simulink model "PSO_controller2"  (R2020a)
settings: Solver=FixedStepAuto  StartTime=0.0  StopTime=Inf  RelTol=1e-3  EnableMultiTasking=on
libraries: c280xlib x11, c2837xDlib x4
settings Model: SimulationMode=external  ExtModeTrigDuration=8  Creator=Jason  LastModifiedBy=Jason
settings SolverCC: AutoInsertRateTranBlk=on
settings OptimizationCC: DefaultUnderspecifiedDataType=single  EnhancedBackFolding=on  PassReuseOutputArgsAs=Individual arguments  MaxStackSize=1024  OptimizeBlockOrder=speed  DifferentSizesBufferReuse=on  OptimizationCustomize=off  DenormalBehavior=FlushToZero  EfficientTunableParamExpr=on
settings DebuggingCC: ParameterTunabilityLossMsg=error
settings HardwareCC: ProdBitPerChar=16  ProdBitPerInt=16  ProdBitPerPointer=32  ProdBitPerSizeT=32  ProdBitPerPtrDiffT=32  ProdLargestAtomicInteger=Integer  ProdLargestAtomicFloat=None  ProdWordSize=16  ProdLongLongMode=on  ProdHWDeviceType=Texas Instruments->C2000
settings RTWCC: SystemTargetFile=ert.tlc  HardwareBoard=TI Delfino F28379D LaunchPad  TLCOptions=-aInlineSetEventsForThisBaseRateFcn=TLC_FALSE -aSuppressMultiTaskScheduler=TLC_FALSE -aRateBasedStepFcn=1  TemplateMakefile=ert_default_tmf  Toolchain=Texas Instruments Code Composer Studio (C2000)
settings CodeAppCC: ForceParamTrailComments=on  IgnoreCustomStorageClasses=off  OperatorAnnotations=on  SimulinkDataObjDesc=on  SFDataObjDesc=on  InsertBlockDesc=on
settings ERTTargetCC: TargetLangStandard=C99 (ISO)  CodeReplacementLibrary=TI C28x  DynamicStringBufferSize=401  SupportVariableSizeSignals=on  ExtModeStaticAllocSize=10000

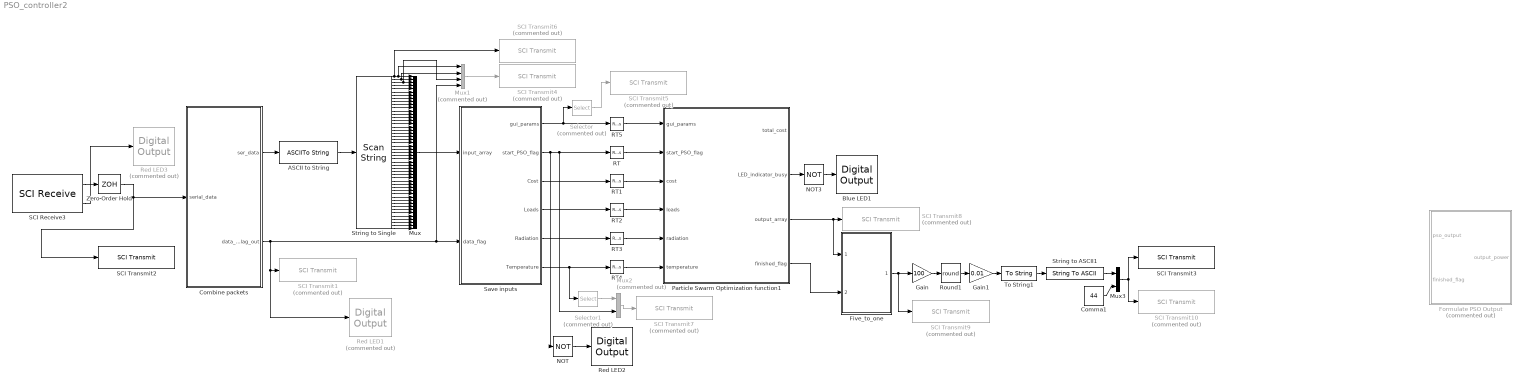
== system PSO_controller2 ==
  ASCII to String : ASCIIToString
  Blue LED1 : c2837xDlib/Digital Output  GPIO_Number=GPIO24~GPIO31  GPIO_Bit0=off  GPIO_BIT0_Toggle=off  GPIO_Bit1=off  GPIO_BIT1_Toggle=off  GPIO_Bit2=off  GPIO_BIT2_Toggle=off  GPIO_Bit3=off  GPIO_BIT3_Toggle=off  GPIO_Bit4=off  GPIO_BIT4_Toggle=off  GPIO_Bit5=off  GPIO_BIT5_Toggle=off  GPIO_Bit6=off  GPIO_BIT6_Toggle=off  GPIO_Bit7=on  GPIO_BIT7_Toggle=off
      settings: SourceProductBaseCode=TIC2000
  Combine packets : MATLAB Function  TreatAsAtomicUnit=on
  Comma1 : Constant  Value=44  OutDataTypeStr=uint8  SampleTime=-1
  Five_to_one : MATLAB Function  TreatAsAtomicUnit=on
  Formulate PSO Output : MATLAB Function  Commented=on  TreatAsAtomicUnit=on
  Gain : Gain  Gain=100
  Gain1 : Gain  Gain=0.01
  Mux : Mux  Inputs=49
  Mux1 : Mux  Commented=on
  Mux2 : Mux  Commented=on  Inputs=2
  Mux3 : Mux  Inputs=2
  NOT : Logic  Operator=NOT  IconShape=distinctive  AllPortsSameDT=off  OutDataTypeStr=boolean
  NOT3 : Logic  Operator=NOT  IconShape=distinctive  AllPortsSameDT=off  OutDataTypeStr=boolean
  Particle Swarm Optimization function1 : MATLAB Function  TreatAsAtomicUnit=on
  RT{,1..5} (6 alike) : RateTransition  OutPortSampleTime=0.1
  Red LED1 : c2837xDlib/Digital Output  Commented=on  GPIO_Number=GPIO32~GPIO39  GPIO_Bit0=off  GPIO_BIT0_Toggle=off  GPIO_Bit1=off  GPIO_BIT1_Toggle=off  GPIO_Bit2=on  GPIO_BIT2_Toggle=off  GPIO_Bit3=off  GPIO_BIT3_Toggle=off  GPIO_Bit4=off  GPIO_BIT4_Toggle=off  GPIO_Bit5=off  GPIO_BIT5_Toggle=off  GPIO_Bit6=off  GPIO_BIT6_Toggle=off  GPIO_Bit7=off  GPIO_BIT7_Toggle=off
      settings: SourceProductBaseCode=TIC2000
  Red LED2 : c2837xDlib/Digital Output  GPIO_Number=GPIO32~GPIO39  GPIO_Bit0=off  GPIO_BIT0_Toggle=off  GPIO_Bit1=off  GPIO_BIT1_Toggle=off  GPIO_Bit2=on  GPIO_BIT2_Toggle=off  GPIO_Bit3=off  GPIO_BIT3_Toggle=off  GPIO_Bit4=off  GPIO_BIT4_Toggle=off  GPIO_Bit5=off  GPIO_BIT5_Toggle=off  GPIO_Bit6=off  GPIO_BIT6_Toggle=off  GPIO_Bit7=off  GPIO_BIT7_Toggle=off
      settings: SourceProductBaseCode=TIC2000
  Red LED3 : c2837xDlib/Digital Output  Commented=on  GPIO_Number=GPIO32~GPIO39  GPIO_Bit0=off  GPIO_BIT0_Toggle=off  GPIO_Bit1=off  GPIO_BIT1_Toggle=off  GPIO_Bit2=on  GPIO_BIT2_Toggle=off  GPIO_Bit3=off  GPIO_BIT3_Toggle=off  GPIO_Bit4=off  GPIO_BIT4_Toggle=off  GPIO_Bit5=off  GPIO_BIT5_Toggle=off  GPIO_Bit6=off  GPIO_BIT6_Toggle=off  GPIO_Bit7=off  GPIO_BIT7_Toggle=off
      settings: SourceProductBaseCode=TIC2000
  Round1 : Rounding  Operator=round
  SCI Receive3 : c280xlib/SCI Receive  sciModule=B  dataHead=''  dataTail=''  dataType=uint8  dataDim=11  initValue=49  errOption=Output the last received value  errValue=0  sampleTime=0.005  outputStatus=on  postInterrupt=off  numFifo=1
      settings: SourceProductBaseCode=TIC2000
  SCI Transmit{1,4..10} (8 alike) : c280xlib/SCI Transmit  Commented=on  sciModule=A  dataHead=''  dataTail=''  postInterrupt=off  numFifo=1
  SCI Transmit2 : c280xlib/SCI Transmit  sciModule=A  dataHead=''  dataTail=''  postInterrupt=off  numFifo=1
  SCI Transmit3 : c280xlib/SCI Transmit  sciModule=B  dataHead=''  dataTail=''  postInterrupt=off  numFifo=1
  Save inputs : MATLAB Function  TreatAsAtomicUnit=on
  Selector : Selector  Commented=on  InputPortWidth=35  IndexOptions=Index vector (dialog)  Indices=[1:4]  OutputSizes=1
  Selector1 : Selector  Commented=on  InputPortWidth=49  IndexOptions=Index vector (dialog)  Indices=[1:3]  OutputSizes=1
  String to ASCII1 : StringToASCII  OutputVectorSize=9
  String to Single : ScanString  Format="\"ff%f,%f,%f,%f,%f,%f,%f,%f,%f,%f,%f,%f,%f,%f,%f,%f,%f,%f,%f,%f,%f,%f,%f,%f,%f,%f,%f,%f,%f,%f,%f,%f,%f,%f,%f,%f,%f,%f,%f,%f,%f,%f,%f,%f,%f,%f,%f,%f,%fE\""
  To String1 : ToString
  Zero-Order Hold : ZeroOrderHold  SampleTime=0.1
  wires:
  SCI Receive3/1 -> Zero-Order Hold/1
  Zero-Order Hold/1 -> Combine packets/1(serial_data), SCI Transmit2/1
  ASCII to String/1 -> String to Single/1
  String to Single/1 -> SCI Transmit6/1, Mux1/1, Mux/1
  String to Single/2 -> Mux1/2, Mux/2
  String to Single/3 -> Mux1/3, Mux/3
  String to Single/4 -> Mux/4
  String to Single/5 -> Mux/5
  String to Single/6 -> Mux/6
  String to Single/7 -> Mux/7
  String to Single/8 -> Mux/8
  String to Single/9 -> Mux/9
  String to Single/10 -> Mux/10
  String to Single/11 -> Mux/11
  String to Single/12 -> Mux/12
  String to Single/13 -> Mux/13
  String to Single/14 -> Mux/14
  String to Single/15 -> Mux/15
  String to Single/16 -> Mux/16
  String to Single/17 -> Mux/17
  String to Single/18 -> Mux/18
  String to Single/19 -> Mux/19
  String to Single/20 -> Mux/20
  String to Single/21 -> Mux/21
  String to Single/22 -> Mux/22
  String to Single/23 -> Mux/23
  String to Single/24 -> Mux/24
  String to Single/25 -> Mux/25
  String to Single/26 -> Mux/26
  String to Single/27 -> Mux/27
  String to Single/28 -> Mux/28
  String to Single/29 -> Mux/29
  String to Single/30 -> Mux/30
  String to Single/31 -> Mux/31
  String to Single/32 -> Mux/32
  String to Single/33 -> Mux/33
  String to Single/34 -> Mux/34
  String to Single/35 -> Mux/35
  String to Single/36 -> Mux/36
  String to Single/37 -> Mux/37
  String to Single/38 -> Mux/38
  String to Single/39 -> Mux/39
  String to Single/40 -> Mux/40
  String to Single/41 -> Mux/41
  String to Single/42 -> Mux/42
  String to Single/43 -> Mux/43
  String to Single/44 -> Mux/44
  String to Single/45 -> Mux/45
  String to Single/46 -> Mux/46
  String to Single/47 -> Mux/47
  String to Single/48 -> Mux/48
  String to Single/49 -> Mux/49
  Mux/1 -> Save inputs/1(input_array)
  Particle Swarm Optimization function1/2(LED_indicator_busy) -> NOT3/1
  NOT3/1 -> Blue LED1/1
  Save inputs/2(start_PSO_flag) -> NOT/1, Mux2/2, RT/1
  Save inputs/3(Cost) -> RT1/1
  Save inputs/4(Loads) -> RT2/1
  Save inputs/5(Radiation) -> RT3/1
  Save inputs/6(Temperature) -> RT4/1, Selector1/1
  SCI Receive3/2 -> Red LED3/1
  Save inputs/1(gui_params) -> Selector/1, RT5/1
  RT5/1 -> Particle Swarm Optimization function1/1(gui_params)
  RT/1 -> Particle Swarm Optimization function1/2(start_PSO_flag)
  RT1/1 -> Particle Swarm Optimization function1/3(cost)
  RT2/1 -> Particle Swarm Optimization function1/4(loads)
  RT3/1 -> Particle Swarm Optimization function1/5(radiation)
  RT4/1 -> Particle Swarm Optimization function1/6(temperature)
  Mux3/1 -> SCI Transmit3/1, SCI Transmit10/1
  Particle Swarm Optimization function1/3(output_array) -> SCI Transmit8/1, Five_to_one/1(input_array_five)
  Combine packets/2(data_status_flag_out) -> Mux1/4, Save inputs/2(data_flag), Red LED1/1, SCI Transmit1/1
  Combine packets/1(ser_data) -> ASCII to String/1
  Mux1/1 -> SCI Transmit4/1
  Selector/1 -> SCI Transmit5/1
  Selector1/1 -> Mux2/1
  Mux2/1 -> SCI Transmit7/1
  Particle Swarm Optimization function1/4(finished_flag) -> Five_to_one/2(finished_flag)
  Gain/1 -> Round1/1
  Five_to_one/1(out_array_one) -> Gain/1, SCI Transmit9/1
  Round1/1 -> Gain1/1
  Gain1/1 -> To String1/1
  To String1/1 -> String to ASCII1/1
  Comma1/1 -> Mux3/2
  String to ASCII1/1 -> Mux3/1
  NOT/1 -> Red LED2/1

== matlab function PSO_controller2/Particle Swarm Optimization function1 ==
  data: total_cost output; gui_params input; start_PSO_flag input; cost input; LED_indicator_busy output; output_array output; loads input; finished_flag output; radiation input; temperature input
% function [total_cost,LED_indicator_busy,output_array,output_array_full,finished_flag,part_table]  = ParticleSwarm_algorithm(gui_params,start_PSO_flag,cost,loads,radiation,temperature)
function [total_cost,LED_indicator_busy,output_array,finished_flag]  = ParticleSwarm_algorithm(gui_params,start_PSO_flag,cost,loads,radiation,temperature)

persistent numParticles maxEpochs currentEpoch currentPar particlesTable neighborIndex EV_bat_n SoC_initial_ev dt Ev_bat_capacity SoC_target_ev Tmax ...
    Tmin T_in_initial V C rho Uwall Uwindow Fwall Fwindow aw Rsej taf_window SC QEC_max QEC_min COP SOC_EV_penalty_multiplier SOC_EV_target_penalty_multiplier ...
    PPEV_diff_penalty_multiplier offset_variable partial_cost_multiplier SoCmax_ev SoCmin_ev lb ub Pmin_ev Pmax_ev Pmax_bat Pmin_bat SoC_initial_bat ...
    SoC_target_bat SoCmax_bat SoCmin_bat bat_capacity bat_n span CostOfPower cSelf cSocial inertia outdoor_temperature solar_radiation heatcool_sign Zeta Qin Qsw Qsg ...
    QEC_diff_penalty_multiplier Tin_penalty_multiplier T t LED_indicator_flag dim1 dim2 dim3 dim4 numVariables tfInvalidMask SOC_bat_penalty_multiplier PBAT_diff_penalty_multiplier home_load ...
    LOAD_equals_penalty_multiplier penaltiesTable minNeighborhoodSize maxParticles maxDimensions output_counter output_delay;



maxParticles = 10;
% maxParticles = 3;
maxDimensions = 13+13+13+13;

% assert(maxEpochs<=1000)

if isempty(LED_indicator_flag)
    LED_indicator_flag = 0;
end


%% Case 1: First run of function, initialize variables
if isempty(currentEpoch)
    
    %     rng shuffle       %MAY NEED TO BE REMOVED
    
    T = 24;
    heatcool_sign = -1;
    output_delay = 1;
    
    % minNeighborhoodSize = max(2,floor(numParticles*0.25)); %0.25 =Minimum adaptive neighborhood size, a scalar from 0 to 1. Default is 0.25.
    minNeighborhoodSize = 2;
    
    
    CostOfPower = single(zeros(1,49));
    home_load = single(zeros(1,49));
    solar_radiation = single(zeros(1,49));
    outdoor_temperature = single(zeros(1,49));

    SOC_EV_penalty_multiplier = 0.5;
    SOC_EV_target_penalty_multiplier = 1.5;
%     PPEV_diff_penalty_multiplier = 0.001;
    PPEV_diff_penalty_multiplier = 0.005;
    
    SOC_bat_penalty_multiplier = 1;
    PBAT_diff_penalty_multiplier = 0.005;
    
    QEC_diff_penalty_multiplier = 0;  % Penalty for large deviations of the QEC
    Tin_penalty_multiplier = 0.6; % Penalty for not maintaining the internal temperature between the desired limits
    
    LOAD_equals_penalty_multiplier = 1; % Penalty for the initial and load shifted loads not having equal sums
    
    offset_variable = 0; %Offset the sum of power rates to avoid reaching negative values
    partial_cost_multiplier = 4;
    cSelf = single(1.496);
    cSocial = single(1.496);
    inertia = single(0.4);%TODO: make inertia vector for each variable
    
    currentEpoch = single(0);
    currentPar = single(0);
    
    
    
    %% Initializations
    numParticles = single(1);
    maxEpochs = single(1);
    
    dt = single(0.5);
    dim1 = single(0);  %EV PSO dimensions
    dim2 = single(0);  %Thermal PSO dimensions
    dim3 = single(0);  %BAT PSO dimensions
    dim4 = single(0);   %Load shifting dimensions
    Pmax_ev = single(0);
    Pmin_ev = single(0);
    EV_bat_n = single(0);
    SoC_initial_ev = single(0);
    SoC_target_ev = single(0);
    Pmax_bat = single(0);
    Pmin_bat = single(0);
    SoC_initial_bat = single(0);
    SoC_target_bat = single(0);
    bat_capacity = single(0);
    bat_n = single(0);
    Tmax = single(0);
    Tmin = single(0);
    T_in_initial = single(0);
    V = single(0);
    C = single(0);
    rho = single(0);
    Uwall = single(0);
    Uwindow = single(0);
    Fwall = single(0);
    Fwindow = single(0);
    aw = single(0);
    Rsej = single(0);
    taf_window = single(0);
    SC = single(0);
    QEC_max = single(0);
    QEC_min = single(0);
    COP = single(0);
    Ev_bat_capacity = single(0);
    t = single(linspace(0,24,(24/0.5)+1));
    
    numVariables = single(maxDimensions);
    tfInvalidMask = single(zeros(10,3*52+1));
    
    Zeta = single((rho*C*V)/(0.5*3600));     %dt is converted to seconds in order to match the rest of the units
    Qin = single(0.2*ones(1,49));
    Qsw = single(aw * Rsej * Uwall * Fwall * solar_radiation);
    Qsg = single(0.001*taf_window * SC * Fwindow * solar_radiation);
    
    SoCmax_ev = single(Ev_bat_capacity*0.9);
    SoCmin_ev = single(Ev_bat_capacity*0.1);
    SoCmax_bat = single(bat_capacity*0.9);
    SoCmin_bat = single(bat_capacity*0.1);
    
    lb = single(zeros(1,maxDimensions));
    ub = single(zeros(1,maxDimensions));
    %     span = single(ub - lb);
    particlesTable = single(zeros(uint8(maxParticles),3*uint8(maxDimensions+1))); %set particlesTable to the largest array size
    output_counter = single(1);
    
    
end

%     %debug
%
%
%     total_cost = 0;
%     LED_indicator_busy = 0;
%     finished_flag = 0;
%     output_array = single(-1*ones(1,4));
%
%
%     %debug

%% Case 2.1: Start optimization (once data has been received), read data and set initial values
if currentEpoch == 0 && start_PSO_flag == 1
    
    
    
    numParticles = gui_params(1);
    maxEpochs = gui_params(2);
    assert(numParticles<=maxParticles)        %Particle matrix will be too big if its more than 11
    
    dim1 = gui_params(3);  %EV PSO dimensions
    dim2 = gui_params(4);  %Thermal PSO dimensions
    dim3 = gui_params(5);  %BAT PSO dimensions
    dim4 = gui_params(6);   %Load shifting dimensions
    assert(dim1<14)
    assert(dim2<14)
    assert(dim3<14)
    assert(dim4<14)
    
    Pmax_ev = gui_params(7);
    Pmin_ev = gui_params(8);
    EV_bat_n = gui_params(9);
    SoC_initial_ev = gui_params(10);
    SoC_target_ev = gui_params(11);
    Pmax_bat = gui_params(12);
    Pmin_bat = gui_params(13);
    SoC_initial_bat = gui_params(14);
    SoC_target_bat = gui_params(15);
    bat_capacity = gui_params(16);
    bat_n = gui_params(17);
    Tmax = gui_params(18);
    Tmin = gui_params(19);
    T_in_initial = gui_params(20);
    V = gui_params(21);
    C = gui_params(22);
    rho = gui_params(23);
    Uwall = gui_params(24);
    Uwindow = gui_params(25);
    Fwall = gui_params(26);
    Fwindow = gui_params(27);
    aw = gui_params(28);
    Rsej = gui_params(29);
    taf_window = gui_params(30);
    SC = gui_params(31);
    QEC_max = gui_params(32);
    QEC_min = gui_params(33);
    COP = gui_params(34);
    Ev_bat_capacity = gui_params(35);
    
    CostOfPower(1:49) = cost(1:49);
    home_load(1:49) = loads(1:49);
    solar_radiation(1:49) = radiation(1:49);
    outdoor_temperature(1:49) = temperature(1:49);
    
    t = single(0:dt:T);
    numVariables = single(dim1+dim2+dim3+dim4);
    assert(numVariables <53)
    tfInvalidMask = single(zeros(numParticles,3*numVariables+1));
    
    Zeta = single((rho*C*V)/(dt*3600));     %dt is converted to seconds in order to match the rest of the units
    Qin = single(0.2*ones(1,length(t)));
    Qsw = single(aw * Rsej * Uwall * Fwall * solar_radiation);
    Qsg = single(0.001*taf_window * SC * Fwindow * solar_radiation);
    
    SoCmax_ev = single(Ev_bat_capacity*0.9);
    SoCmin_ev = single(Ev_bat_capacity*0.1);
    SoCmax_bat = single(bat_capacity*0.9);
    SoCmin_bat = single(bat_capacity*0.1);
    
    Load_shifting_min = 0.7;
    Load_shifting_max = 1.3;
    
    
    
    if QEC_min == 0 && QEC_max == 0     %No heat system or load system
        QEC_diff_penalty_multiplier = 0;
        Tin_penalty_multiplier = 0;
        LOAD_equals_penalty_multiplier = 0;
        Load_shifting_min = 0;
        Load_shifting_max = 0;
    end
    
    
    lb = single([Pmin_ev*ones(1,dim1) QEC_min*ones(1,dim2) Pmin_bat*ones(1,dim3) Load_shifting_min*ones(1,dim4)]);
    ub = single([Pmax_ev*ones(1,dim1) QEC_max*ones(1,dim2) Pmax_bat*ones(1,dim3) Load_shifting_max*ones(1,dim4)]);
    span = single(ub - lb);
    
    %     particlesTable = single(zeros(uint8(numParticles),3*uint8(numVariables+1))); %kathe numVariables plithos timon, gia kathe dianusma (current pos, best pos, velocity)
    particlesTable(:,1:numVariables) = repmat(lb,numParticles,1) + repmat(span,numParticles,1) .* rand(numParticles,numVariables);
    particlesTable(:,numVariables+2:numVariables+2+numVariables-1) = particlesTable(:,1:numVariables);
    % Initialize velocities by randomly sampling over the smaller of options.InitialSwarmSpan or ub-lb. Note that min will be InitialSwarmSpan if either lb or ub is not finite.
    vmax = single(span);
    particlesTable(:,2*numVariables+2:2*numVariables+2+numVariables-1) = repmat(-vmax,numParticles,1) + ...
        repmat(2*vmax,numParticles,1) .* rand(numParticles,numVariables);
    
    currentPar = currentPar + 1;
    
    % EV Calculations
    [PPEV,state_of_charge_ev] = EV_Calculations(dt,T,dim1,currentPar,particlesTable,EV_bat_n,SoC_initial_ev);
    
    % Heat System Calculations
    [QEC,indoor_temperature] = Thermal_Calculations(dt,T,dim1,dim2,currentPar,particlesTable,COP,T_in_initial,heatcool_sign,Zeta,Uwall,Uwindow,Fwall,Fwindow,outdoor_temperature,Qin,Qsw,Qsg);
    
    % BAT Calculations
    [PBAT,state_of_charge_bat] = Bat_Calculations(dt,T,dim1,dim2,dim3,currentPar,particlesTable,bat_n,SoC_initial_bat);
    
    % LOAD Calculations
    [PLOAD] = Load_Calculations(dt,T,dim1,dim2,dim3,dim4,currentPar,particlesTable,home_load);
    
    % EV Penalty
    [SOC_ev_penalty,SOC_ev_target_penalty,PPEV_diff_penalty] = EV_Penalties(state_of_charge_ev,SoCmax_ev,SoCmin_ev,PPEV,SoC_target_ev) ;
    
    % Heat System Penalty
    [Tin_penalty,QEC_diff_penalty] = Thermal_Penalties(QEC,indoor_temperature,Tmax,Tmin);
    
    % BAT Penalty
    [SOC_bat_penalty,PBAT_diff_penalty] = Bat_Penalties(state_of_charge_bat,SoCmax_bat,SoCmin_bat,PBAT,SoC_target_bat) ;
    
    % LOAD penalty
    [Load_equals_penalty] = Load_Penalties(PLOAD,home_load);
    
    % Cost Calculations
    cost_partial = single(sum((PPEV+abs(QEC)+PBAT+PLOAD').*CostOfPower)*dt);
    total_cost =single((SOC_EV_target_penalty_multiplier * SOC_ev_target_penalty + SOC_EV_penalty_multiplier * SOC_ev_penalty + ...
        PPEV_diff_penalty_multiplier * PPEV_diff_penalty + QEC_diff_penalty_multiplier*QEC_diff_penalty + Tin_penalty_multiplier*Tin_penalty + ...
        SOC_bat_penalty * SOC_bat_penalty_multiplier + PBAT_diff_penalty * PBAT_diff_penalty_multiplier + Load_equals_penalty * LOAD_equals_penalty_multiplier)+ ...
        (partial_cost_multiplier*(offset_variable+cost_partial)));
    
    particlesTable(currentPar,numVariables+1) = total_cost; %fval of previous particle stored as the best value of this particle (since it is the first time that it gets a value)
    

    
    %Finalize initialization, start main loop
    if currentPar == numParticles
        currentEpoch =single(1);
        currentPar = single(0);
        
    end
    
    LED_indicator_busy = 0;
    finished_flag = single(0);

    output_array = single(-1*ones(1,5));
    output_array(1) = currentPar;
    output_array(2) = numParticles;
    output_array(3) = maxEpochs;
    output_array(4) = dim1;
    output_array(5) = dim2;
    
    %% Case 2.2: Main loop of optimization
elseif currentEpoch <= maxEpochs && start_PSO_flag == 1
    
    
    
    if LED_indicator_flag == 0
        LED_indicator_flag = 1;
        LED_indicator_busy = 1;
    else
        LED_indicator_flag = 0;
        LED_indicator_busy = 0;
    end
    
    currentPar = currentPar + 1;
    
    %     part_table = particlesTable(currentPar,1:157)';
    %     part_table(1)=single(222222);
    %     part_table(2)=particlesTable(currentPar,53);
    
    if currentPar == 1
        
        % Generate a random neighborhood for each particle that includes the particle itself
        neighborIndex = zeros(numParticles, minNeighborhoodSize);
        neighborIndex(:, 1) = 1:numParticles; % First neighbor is self
        for i = 1:numParticles
            % Determine random neighbors that exclude the particle itself, which is (numParticles-1) particles
            neighbors = randperm(numParticles-1, minNeighborhoodSize-1);
            % Add 1 to indices that are >= current particle index
            iShift = neighbors >= i;
            neighbors(iShift) = neighbors(iShift) + 1;
            neighborIndex(i,2:end) = neighbors;
        end
        
        randSelf = rand(numParticles, numVariables);
        randSocial = rand(numParticles, numVariables);
        
        % Update the velocities
        
        temp1 = inertia*particlesTable(:,2*numVariables+2:2*numVariables+2+numVariables-1);
        temp2 = cSelf*randSelf.*(particlesTable(:,numVariables+2:numVariables+2+numVariables-1)-particlesTable(:,1:numVariables));
        %  temp3 =  cSocial*randSocial.*(particlesTable(bestNeighborIndex,numVariables+2:numVariables+2+numVariables-1)-particlesTable(:,1:numVariables))
        
        temp3 =  cSocial*randSocial.*(particlesTable(neighborIndex(:,2:end),numVariables+2:numVariables+2+numVariables-1)-particlesTable(:,1:numVariables));
        newVelocities =  temp1 + ...
            temp2 + ... %%thesi poy eixe kaluteri timi - current thesi
            temp3;
        
        particlesTable(:,2*numVariables+2:2*numVariables+2+numVariables-1) = newVelocities;
        
        % Update the positions
        newPopulation = particlesTable(:,1:numVariables) + particlesTable(:,2*numVariables+2:2*numVariables+2+numVariables-1);
        
        tfInvalid=zeros(numParticles,numVariables);
        for i=1:numParticles
            tfInvalid(i,:) = newPopulation(i,:) < lb;
        end
        tfInvalidMask(:,2*numVariables+2:end) = tfInvalid;
        mask = (tfInvalidMask==1);
        
        
        if any(any(tfInvalid))
            for y=1:numVariables
                for i=1:numParticles
                    if tfInvalid(i,y)==1
                        newPopulation(i,y)= lb(y);
                    end
                end
            end
            particlesTable(mask) = 0;
        end
        
        
        tfInvalid=zeros(numParticles,numVariables);
        for i=1:numParticles
            tfInvalid(i,:) = newPopulation(i,:) > ub;
        end
        tfInvalidMask(:,2*numVariables+2:end) = tfInvalid;
        mask = (tfInvalidMask==1);
        if any(any(tfInvalid))
            for y=1:numVariables
                for i=1:numParticles
                    if tfInvalid(i,y)==1
                        newPopulation(i,y)= ub(y);
                    end
                end
            end
            particlesTable(mask) = 0;
        end
        particlesTable(:,1:numVariables) = newPopulation;
    end
    
    %     part_table(3)=particlesTable(currentPar,53);
    
    
    % EV Calculations
    [PPEV,state_of_charge_ev] = EV_Calculations(dt,T,dim1,currentPar,particlesTable,EV_bat_n,SoC_initial_ev);
    
    % Thermal Calculations
    [QEC,indoor_temperature] = Thermal_Calculations(dt,T,dim1,dim2,currentPar,particlesTable,COP,T_in_initial,heatcool_sign,Zeta,Uwall,Uwindow,Fwall,Fwindow,outdoor_temperature,Qin,Qsw,Qsg);
    
    % BAT Calculations
    [PBAT,state_of_charge_bat] = Bat_Calculations(dt,T,dim1,dim2,dim3,currentPar,particlesTable,bat_n,SoC_initial_bat);
    
    % LOAD Calculations
    [PLOAD] = Load_Calculations(dt,T,dim1,dim2,dim3,dim4,currentPar,particlesTable,home_load);
    
    % EV Penalty
    [SOC_ev_penalty,SOC_ev_target_penalty,PPEV_diff_penalty] = EV_Penalties(state_of_charge_ev,SoCmax_ev,SoCmin_ev,PPEV,SoC_target_ev) ;
    
    % Heat System Penalty
    [Tin_penalty,QEC_diff_penalty] = Thermal_Penalties(QEC,indoor_temperature,Tmax,Tmin);
    
    % BAT Penalty
    [SOC_bat_penalty,PBAT_diff_penalty] = Bat_Penalties(state_of_charge_bat,SoCmax_bat,SoCmin_bat,PBAT,SoC_target_bat) ;
    
    % LOAD penalty
    [Load_equals_penalty] = Load_Penalties(PLOAD,home_load);
    
    %% ------------- Cost Calculations -------------
    
    if QEC_min == 0 && QEC_max == 0     %No heat system or load system
        cost_partial = single(sum((PPEV+PBAT).*CostOfPower)*dt);
    else
        cost_partial = single(sum((PPEV+abs(QEC)+PBAT+PLOAD').*CostOfPower)*dt);
    end
    total_cost =single((SOC_EV_target_penalty_multiplier * SOC_ev_target_penalty + SOC_EV_penalty_multiplier * SOC_ev_penalty + ...
        PPEV_diff_penalty_multiplier * PPEV_diff_penalty + QEC_diff_penalty_multiplier*QEC_diff_penalty + Tin_penalty_multiplier*Tin_penalty + ...
        SOC_bat_penalty * SOC_bat_penalty_multiplier + PBAT_diff_penalty * PBAT_diff_penalty_multiplier + Load_equals_penalty * LOAD_equals_penalty_multiplier)+ ...
        (partial_cost_multiplier*(offset_variable+cost_partial)));
    
    %     part_table(4)=particlesTable(currentPar,53);
    %     part_table(5)=total_cost;
    
    
    if total_cost < particlesTable(currentPar,numVariables+1)
        
        particlesTable(currentPar,numVariables+1) = total_cost;
        particlesTable(currentPar,numVariables+2:numVariables+2+numVariables-1) = particlesTable(currentPar,1:numVariables);
        
        
        %         %DEBUGGING, REMOVE LATER
        %         penaltiesTable(currentPar,1) = SOC_EV_target_penalty_multiplier * SOC_ev_target_penalty;
        %         penaltiesTable(currentPar,2) = SOC_EV_penalty_multiplier * SOC_ev_penalty;
        %         penaltiesTable(currentPar,3) = PPEV_diff_penalty_multiplier * PPEV_diff_penalty;
        %         penaltiesTable(currentPar,4) = QEC_diff_penalty_multiplier*QEC_diff_penalty;
        %         penaltiesTable(currentPar,5) = Tin_penalty_multiplier*Tin_penalty;
        %         penaltiesTable(currentPar,6) = SOC_bat_penalty * SOC_bat_penalty_multiplier;
        %         penaltiesTable(currentPar,7) = PBAT_diff_penalty * PBAT_diff_penalty_multiplier;
        %         penaltiesTable(currentPar,8) = Load_equals_penalty * LOAD_equals_penalty_multiplier;
        %         penaltiesTable(currentPar,10) = cost_partial;
        %         penaltiesTable(currentPar,9)= (SOC_EV_target_penalty_multiplier * SOC_ev_target_penalty + SOC_EV_penalty_multiplier * SOC_ev_penalty + ...
        %         PPEV_diff_penalty_multiplier * PPEV_diff_penalty + QEC_diff_penalty_multiplier*QEC_diff_penalty + Tin_penalty_multiplier*Tin_penalty + ...
        %         SOC_bat_penalty * SOC_bat_penalty_multiplier + PBAT_diff_penalty * PBAT_diff_penalty_multiplier + Load_equals_penalty * LOAD_equals_penalty_multiplier);
        % %         penaltiesTable(10)= partial_cost_multiplier*(offset_variable+cost_partial);
        %
        %
    end
    
    %     part_table(6)=particlesTable(currentPar,53);
    %     part_table(7)=total_cost;
    
    output_array = single(-2*ones(1,5));
    
    finished_flag = single(0);
    %     part_table = particlesTable(currentPar,1:157)';
    
    %End of current epoch
    if currentPar == numParticles
        currentEpoch = currentEpoch + 1;
        
%         if currentEpoch > maxEpochs 
%             particlesTable(:,numVariables+2:numVariables+numVariables+1) = 100.*(particlesTable(:,numVariables+2:numVariables+numVariables+1));
%             particlesTable(:,numVariables+2:numVariables+numVariables+1) = round(particlesTable(:,numVariables+2:numVariables+numVariables+1));
%             particlesTable(:,numVariables+2:numVariables+numVariables+1) = (particlesTable(:,numVariables+2:numVariables+numVariables+1)/100);
%         end
        
        currentPar = single(0);
        return;
        %End of current particle
    elseif currentPar>=1 && currentPar<numParticles
        return;
    else %Should never reach here
        error('Particle Loop Error')
    end
    
    
    %% Case 2.3: Optimization ended, and no new data has been sent - Output power arrays
elseif start_PSO_flag == 1  %end of PSO calculations
    
    [total_cost,i_min_cost] = min(particlesTable(1:numParticles,numVariables+1));
    LED_indicator_busy = 1;
    
    finished_flag = single(1);
    
    %% ------------- Debug Calculations and plots -------------
    
    particlesTable(:,1:numVariables) = particlesTable(:,numVariables+2:numVariables+numVariables+1);
    
    
    [PPEV,state_of_charge_ev] = EV_Calculations(dt,T,dim1,i_min_cost,particlesTable,EV_bat_n,SoC_initial_ev);
    [QEC,indoor_temperature] = Thermal_Calculations(dt,T,dim1,dim2,i_min_cost,particlesTable,COP,T_in_initial,heatcool_sign,Zeta,Uwall,Uwindow,Fwall,Fwindow,outdoor_temperature,Qin,Qsw,Qsg);
    [PBAT,state_of_charge_bat] = Bat_Calculations(dt,T,dim1,dim2,dim3,i_min_cost,particlesTable,bat_n,SoC_initial_bat);
    [PLOAD] = Load_Calculations(dt,T,dim1,dim2,dim3,dim4,i_min_cost,particlesTable,home_load);
    
    PPEV(end)=0;
    PBAT(end)=0;
    
%     
    output_array_temp = single([1111111 PPEV(1:49) 2222222 PBAT(1:49) 3333333 QEC(1:49) 4444444 indoor_temperature(1:49) ...
        5555555 state_of_charge_ev(1:49) 6666666 state_of_charge_bat(1:49) 7777777 PLOAD(1:49)']);
%     debug_array = [1 2 3 4 5 6 7 8 9 10 11 12 13 14 15 16 17 18 19 20 21 22 23 24 25 26 27 28 29 30 31 32 33 34 35 36 37 38 39 40 41 42 43 44 45 46 47 48 49];
%     output_array_temp = single([1111111 debug_array 2222222 debug_array 3333333 debug_array 4444444 debug_array ...
%         5555555 debug_array 6666666 debug_array 7777777 debug_array]);
%     
    output_array = single(-4*ones(1,5));
    output_array(1) = output_array_temp(output_counter);
    output_array(2) = output_array_temp(output_counter+1);
    output_array(3) = output_array_temp(output_counter+2);
    output_array(4) = output_array_temp(output_counter+3);
    output_array(5) = output_array_temp(output_counter+4);
    
        output_delay = output_delay + 1;
        if output_delay > 5
            output_counter = output_counter + 5;
            output_delay = 1;
        end
    
%     output_counter = output_counter + 5;
    
    
    if output_counter > size(output_array_temp)
        output_counter = single(1);
    end
    
    
    %% Case 2.4: Optimization ended, new data is being sent
else
    total_cost = single(100000);
    LED_indicator_busy = 0;
    finished_flag = single(0);
    %     part_table = single(38*ones(1,157)');
    output_array = single(-3*ones(1,5));
    
    currentEpoch = single(0);
    
end

end



function [PPEV,state_of_charge_ev] = EV_Calculations(dt,T,dim1,currentPar,particlesTable,EV_bat_n,SoC_initial_ev)

PPEV_not_interp = single(particlesTable(currentPar,1:dim1));
% PPEV = single(interp1(linspace(0,T,dim1),PPEV_not_interp,linspace(0,T,(T/dt)+1),'spline'));
PPEV = single(interp1(0:2:T,PPEV_not_interp,0:0.5:T,'spline'));

PPEV_actual = single(zeros(1,length(PPEV))');
for z=1:length(PPEV_actual)
    if PPEV(z)>=0
        PPEV_actual(z)=PPEV(z)*EV_bat_n;
    else
        PPEV_actual(z)=PPEV(z)/EV_bat_n;
    end
end

state_of_charge_ev = single(zeros(1,length(PPEV)));
state_of_charge_ev(1)=SoC_initial_ev;
state_of_charge_ev(2:end)=SoC_initial_ev+cumsum(PPEV_actual(1:end-1))*dt;

end
function [QEC,indoor_temperature] = Thermal_Calculations(dt,T,dim1,dim2,currentPar,particlesTable,COP,T_in_initial,heatcool_sign,Zeta,Uwall,Uwindow,Fwall,Fwindow,outdoor_temperature,Qin,Qsw,Qsg)

QEC_not_interp = single(particlesTable(currentPar,dim1+1:dim1+dim2));  % TODO Fix number of variables once you add more power arrays to calculate
QEC = single(interp1(linspace(0,T,dim2),QEC_not_interp,linspace(0,T,(T/dt)+1),'spline'));
QEC_thermal = single(QEC*COP);

indoor_temperature=single(zeros(1,length(QEC_thermal)));
indoor_temperature(1) =T_in_initial;

for i=2:length(QEC)
    indoor_temperature(i) = indoor_temperature(i-1) + heatcool_sign*QEC_thermal(i-1)/Zeta + ...
        (Uwall*Fwall*(outdoor_temperature(i-1)-indoor_temperature(i-1))+ ...
        Uwindow*Fwindow*(outdoor_temperature(i-1)-indoor_temperature(i-1))+ ...
        Qin(i-1)+Qsw(i-1)+Qsg(i-1))/Zeta;
end

end
function [PBAT,state_of_charge_bat] = Bat_Calculations(dt,T,dim1,dim2,dim3,currentPar,particlesTable,bat_n,SoC_initial_bat)

PBAT_not_interp = single(particlesTable(currentPar,dim1+dim2+1:dim1+dim2+dim3));
PBAT = single(interp1(linspace(0,T,dim3),PBAT_not_interp,linspace(0,T,(T/dt)+1),'spline'));

PBAT_actual = zeros(1,length(PBAT))';
for z=1:length(PBAT_actual)
    if PBAT(z)>=0
        PBAT_actual(z)=PBAT(z)*bat_n;
    else
        PBAT_actual(z)=PBAT(z)/bat_n;
    end
end

state_of_charge_bat = single(zeros(1,length(PBAT)));
state_of_charge_bat(1)=SoC_initial_bat;
state_of_charge_bat(2:end) = SoC_initial_bat + cumsum(PBAT_actual(1:end-1))*dt;

end
function [PLOAD] = Load_Calculations(dt,T,dim1,dim2,dim3,dim4,currentPar,particlesTable,home_load)

PLOAD_shifting_not_interp = single(particlesTable(currentPar,dim1+dim2+dim3+1:dim1+dim2+dim3+dim4));
PLOAD_shifting = single(interp1(linspace(0,T,dim4),PLOAD_shifting_not_interp,linspace(0,T,(T/dt)+1),'spline'));
PLOAD = (PLOAD_shifting.*home_load)';

end
function [SOC_ev_penalty,SOC_ev_target_penalty,PPEV_diff_penalty] = EV_Penalties(state_of_charge_ev,SoCmax_ev,SoCmin_ev,PPEV,SoC_target_ev)
SOC_ev_penalty = single(0);
for i=1:length(state_of_charge_ev)
    if state_of_charge_ev(i)>SoCmax_ev
        SOC_ev_penalty = SOC_ev_penalty + (state_of_charge_ev(i) - SoCmax_ev);
    elseif  state_of_charge_ev(i)<SoCmin_ev
        SOC_ev_penalty = SOC_ev_penalty + (SoCmin_ev - state_of_charge_ev(i));
    end
end
SOC_ev_target_penalty= single(abs(state_of_charge_ev(end)-SoC_target_ev));

PPEV_diff_penalty = single(sum(abs(diff(PPEV))));
end
function [Tin_penalty,QEC_diff_penalty] = Thermal_Penalties(QEC,indoor_temperature,Tmax,Tmin)

Tin_penalty = single(0);
for i=1:length(QEC)
    if indoor_temperature(i)>Tmax(1)
        Tin_penalty = Tin_penalty + (indoor_temperature(i) - Tmax(1));
    elseif  indoor_temperature(i)<Tmin(1)
        Tin_penalty = Tin_penalty + (Tmin(1) - indoor_temperature(i));
    end
end
QEC_diff_penalty=single(sum(abs(diff(QEC))));
end
function [SOC_bat_penalty,PBAT_diff_penalty] = Bat_Penalties(state_of_charge_bat,SoCmax_bat,SoCmin_bat,PBAT,SoC_target_bat)
SOC_bat_penalty = single(0);
for i=1:length(PBAT)
    if state_of_charge_bat(i)>SoCmax_bat
        SOC_bat_penalty = SOC_bat_penalty + (state_of_charge_bat(i) - SoCmax_bat);
    elseif  state_of_charge_bat(i)<SoCmin_bat
        SOC_bat_penalty = SOC_bat_penalty + (SoCmin_bat - state_of_charge_bat(i));
    end
end
SOC_bat_penalty = SOC_bat_penalty + abs(state_of_charge_bat(end)-SoC_target_bat);
PBAT_diff_penalty=sum(abs(diff(PBAT)    )   );

end
function [Load_equals_penalty] = Load_Penalties(PLOAD,home_load)
Load_equals_penalty = abs(sum(PLOAD)-sum(home_load));
end

== matlab function PSO_controller2/Five_to_one ==
  data: input_array_five input; out_array_one output; finished_flag input
function out_array_one = five_to_one(input_array_five,finished_flag)

persistent counter

if isempty(counter)
    counter = single(0);
end

if finished_flag == 1
    counter=counter+1;
    out_array_one = input_array_five(counter);
    if counter == 5
        counter = single(0);
    end

else
    out_array_one = single(-88);
end

== matlab function PSO_controller2/Formulate PSO Output ==
  data: pso_output input; output_power output single size=1 2; finished_flag input
function output_power = Formulate_output(pso_output,finished_flag)

persistent i output_array counter
if isempty(i)
    i = single(0);
    counter = single(0);
    output_array = single(zeros(1,2));
end

if finished_flag == 1
    i = i + single(1);

    if i == 200 %every 20 seconds
        
        output_array(1) = pso_output(1+counter);
        output_array(2) = pso_output(50+counter);
        counter = counter+ single(1);
        if counter == 49
            counter = single(0);
        end
        i = single(0);
        
    end
end
output_power = output_array;

== matlab function PSO_controller2/Combine packets ==
  data: serial_data input; ser_data output; data_status_flag_out output
function [ser_data,data_status_flag_out] = combine_packets(serial_data)

% serial_data[] is sent in packets of 50 ASCII characters
% data_status_flag -> -1: no data, 0: receiving data, 1: finished GUI,
% 2: finished Cost, 3: finished Loads, 4: finished Radiation,
% 5: finished Temperature, 6: wrong data

persistent counter data data_status_flag

if isempty(counter)
    counter = single(0);
    data = uint8(zeros(1,400));
    data_status_flag = single(-1);
end


if serial_data(1) == 'A' && serial_data(2) == 'S' %Start Signal
    counter = single(1);
    data_status_flag = single(0);
end

if counter > 0
    
    if serial_data(1) == counter+64
            data((counter-1)*10+1:(counter-1)*10+10) = serial_data(2:11);
            counter = counter + 1;
    end
    
    
    if counter == 41   %Full 400 bytes received
        counter = single(0);
        
        if data(2) == 'G'
            data_status_flag = single(1);
        elseif data(2) == 'C'
            data_status_flag = single(2);
        elseif data(2) == 'L'
            data_status_flag = single(3);
        elseif data(2) == 'R'
            data_status_flag = single(4);
        elseif data(2) == 'T'
            data_status_flag = single(5);
        else %error
            data_status_flag = single(6);
        end
        data(1) = 'f';
        data(2) = 'f';
    end
end


ser_data = data;
data_status_flag_out = data_status_flag;

== matlab function PSO_controller2/Save inputs ==
  data: input_array input; gui_params output size=1 35; data_flag input; start_PSO_flag output; Cost output size=1 49; Loads output size=1 49; Radiation output size=1 49; Temperature output size=1 49
function [gui_params,start_PSO_flag,Cost,Loads,Radiation,Temperature]= save_inputs(input_array,data_flag)

% data_flag -> -1: no data, 0: receiving data, 1: finished GUI,
% 2: finished Cost, 3: finished Loads, 4: finished Radiation,
% 5: finished Temperature, 6: wrong data

persistent gui_par PSO_flag Cost_array Loads_array Radiation_array Temperature_array

if isempty(gui_par)
    gui_par = single(zeros(1,35));
    Cost_array = single(zeros(1,49));
    Loads_array = single(zeros(1,49));
    Radiation_array = single(zeros(1,49));
    Temperature_array = single(zeros(1,49));
end

if data_flag == 1
    gui_par(1:35) = input_array(1:35);
    PSO_flag = single(0);
elseif data_flag == 2
    Cost_array(1:49) = input_array;
    PSO_flag = single(0);
elseif data_flag == 3
    Loads_array(1:49) = input_array;
    PSO_flag = single(0);
elseif data_flag == 4
    Radiation_array(1:49) = input_array;
    PSO_flag = single(0);
elseif data_flag == 5
    Temperature_array(1:49) = input_array;
    PSO_flag = single(1);
else
    PSO_flag = single(0);
end



gui_params = gui_par;
start_PSO_flag = PSO_flag;
Cost = Cost_array;
Loads = Loads_array;
Radiation = Radiation_array;
Temperature = Temperature_array;
